simulink model "iros2018_AoA"  (R2017b)
settings: Solver=FixedStepAuto  StartTime=0.0  StopTime=sim_time  FixedStep=1e-5  MaxStep=1e-3  MinStep=1e-19
values from neighbouring files (symbols this model uses):
  g = 9.8    [parameters.m]    (also in parameters.mat)
  I_B = [I_B_x 0 0; 0 I_B_y 0; 0 0 I_B_z]    [parameters.m]    (also in parameters.mat = [5e-10  0  0; 0  5e-10  0; 0  0  1e-09])
  m = 60e-6    (= 6e-05)    [parameters.m]    (also in parameters.mat)
  M2 = [0                  sin(angle)      0               -sin(angle) ... (first row only)    [parameters.m]    (also in parameters.mat = [0 0 1 0 -0.01 0.01 0 0 1 0 -0.01 -0.01 ... (24 elements, 6x)
  M_pitch = -1*[1,1,-1,-1]'    [parameters.m]    (also in parameters.mat = [-1 -1 1 1])
  M_roll = [1,-1,-1,1]'    [parameters.m]    (also in parameters.mat = [1 -1 -1 1])
  M_z = [1,1,1,1]'    [parameters.m]    (also in parameters.mat = [1 1 1 1])
  quad = struct('g',g,'M',m)    [LinearDroneAndPolePlaceControl_ME231b.m]    (also in PolePlacement_DesiredState.m)
  state_des = [0; 0; -.1 ; 0; .00; .00; 0; 0; 0; 0; 0; 0]    [LinearDroneAndPolePlaceControl_ME231b.m]    (also in PolePlacement_DesiredState.m = [0; 0; .015; 0; .00; .00; 0; 0; 0; 0; 0; 0])
  XYZ_initial_condition = [0.0; 0.0; 0.0]    [LinearDroneAndPolePlaceControl_ME231b.m]    (also in PolePlacement_DesiredState.m)
libraries: simulink x15, aerolibutil x2
settings Model: Creator=cbschindler  LastModifiedBy=nato
settings SolverCC: MaxConsecutiveMinStep=15  SolverResetMethod=Robust
settings DataIOCC: LimitDataPoints=on  SaveFormat=Array
settings OptimizationCC: LifeSpan=inf
settings DebuggingCC: ModelReferenceExtraNoncontSigs=none  SFUnexpectedBacktrackingDiag=warning  SFNoUnconditionalDefaultTransitionDiag=warning  SFExecutionAtInitializationDiag=none
settings HardwareCC: ProdBitPerPointer=32  ProdBitPerSizeT=32  ProdBitPerPtrDiffT=32  ProdLargestAtomicFloat=None  ProdIntDivRoundTo=Undefined  ProdEndianess=Unspecified  ProdWordSize=32  ProdHWDeviceType=32-bit Generic
settings ModelReferenceCC: PropagateSignalLabelsOutOfModel=off
settings CodeAppCC: StateflowObjectComments=on
settings GRTTargetCC: TargetLangStandard=C89/C90 (ANSI)  GeneratePreprocessorConditionals=Disable all
settings ConfigComp: CovMetricSettings=dw  CovHtmlReporting=on  CovSaveCumulativeToWorkspaceVar=on  CovSaveSingleToWorkspaceVar=on  CovExternalEMLEnable=off

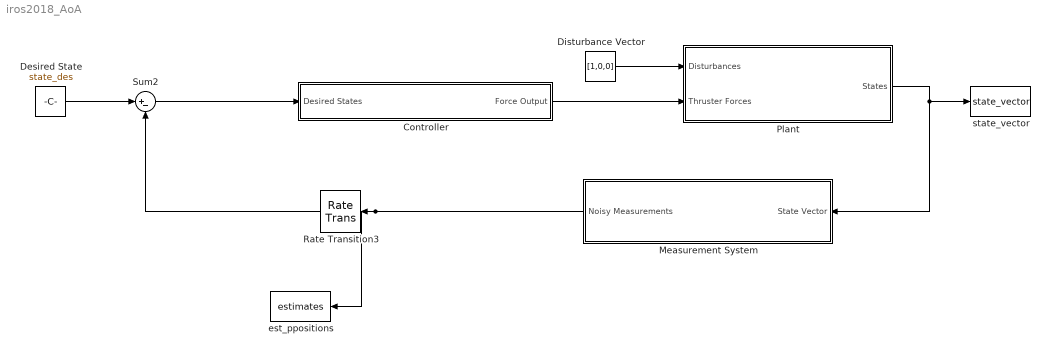
== system iros2018_AoA ==
  Controller : Subsystem
  Desired State : Constant  Value=state_des
  Disturbance Vector : Constant  Value=[1,0,0]
  Measurement System : Subsystem
  Plant : Subsystem
  Rate Transition3 : RateTransition  OutPortSampleTime=0.005
  Sum2 : Sum  Inputs=|+-
  est_ppositions : ToWorkspace  VariableName=estimates  SaveFormat=Timeseries  SampleTime=-1
  state_vector : ToWorkspace  VariableName=state_vector  SaveFormat=Timeseries  SampleTime=-1
  wires:
  Desired State/1 -> Sum2/1
  Rate Transition3/1 -> Sum2/2
  Measurement System/1(Noisy Measurements) -> est_ppositions/1, Rate Transition3/1
  Sum2/1 -> Controller/1(Desired States)
  Plant/1("States ") -> state_vector/1, Measurement System/1("State Vector ")
  Controller/1(Force Output) -> Plant/2(Thruster Forces)
  Disturbance Vector/1 -> Plant/1(Disturbances)

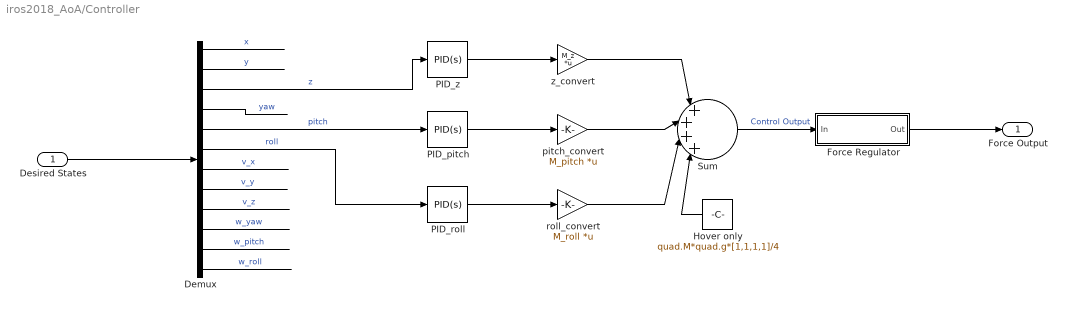
== system iros2018_AoA/Controller ==
  Desired States : Inport
  Demux : Demux  Outputs=12
  Force Regulator : Subsystem
  Hover only : Constant  Value=quad.M*quad.g*[1,1,1,1]/4
  PID_pitch : simulink/Continuous/PID Controller  Controller=PID  TimeDomain=Continuous-time  SampleTime=-1  IntegratorMethod=Forward Euler  FilterMethod=Forward Euler  Form=Parallel  UseFilter=on  ControllerParametersSource=internal  P=0.00000843627433781939  I=.00000750505503699886  D=9.57966094473437e-07  N=33.5514195440974  InitialConditionSource=internal  InitialConditionForIntegrator=0  InitialConditionForFilter=0  ExternalReset=none  LimitOutput=off  UpperSaturationLimit=inf  LowerSaturationLimit=-inf  LinearizeAsGain=on  AntiWindupMode=none  Kb=1  TrackingMode=off  Kt=1  PParamMin=[]  PParamMax=[]  IParamMin=[]  IParamMax=[]  DParamMin=[]  DParamMax=[]  NParamMin=[]  NParamMax=[]  KbParamMin=[]  KbParamMax=[]  KtParamMin=[]  KtParamMax=[]  POutMin=[]  POutMax=[]  IOutMin=[]  IOutMax=[]  DOutMin=[]  DOutMax=[]  NOutMin=[]  NOutMax=[]  KbOutMin=[]  KbOutMax=[]  KtOutMin=[]  KtOutMax=[]  IntegratorOutMin=[]  IntegratorOutMax=[]  FilterOutMin=[]  FilterOutMax=[]  SumOutMin=[]  SumOutMax=[]  SumI1OutMin=[]  SumI1OutMax=[]  SumI2OutMin=[]  SumI2OutMax=[]  SumI3OutMin=[]  SumI3OutMax=[]  SumDOutMin=[]  SumDOutMax=[]  SaturationOutMin=[]  SaturationOutMax=[]  IntegratorContinuousStateAttributes=''  IntegratorStateMustResolveToSignalObject=off  IntegratorRTWStateStorageClass=Auto  FilterContinuousStateAttributes=''  FilterStateMustResolveToSignalObject=off  FilterRTWStateStorageClass=Auto  DifferentiatorICPrevScaledInput=0  DifferentiatorOutMin=[]  DifferentiatorOutMax=[]  InitialConditionSetting=State (most efficient)  FilterDiffOutCoefMin=[]  FilterDiffOutCoefMax=[]  SumDenOutMin=[]  SumDenOutMax=[]  SumNumOutMin=[]  SumNumOutMax=[]  ReciprocalOutMin=[]  ReciprocalOutMax=[]  DivideOutMin=[]  DivideOutMax=[]  TunerSelectOption=Transfer Function Based (PID Tuner App)
  PID_roll : simulink/Continuous/PID Controller  Controller=PID  TimeDomain=Continuous-time  SampleTime=-1  IntegratorMethod=Forward Euler  FilterMethod=Forward Euler  Form=Parallel  UseFilter=on  ControllerParametersSource=internal  P=0.00000843627433781939  I=.00000750505503699886  D=9.57966094473437e-07  N=33.5514195440974  InitialConditionSource=internal  InitialConditionForIntegrator=0  InitialConditionForFilter=0  ExternalReset=none  LimitOutput=off  UpperSaturationLimit=inf  LowerSaturationLimit=-inf  LinearizeAsGain=on  AntiWindupMode=none  Kb=1  TrackingMode=off  Kt=1  PParamMin=[]  PParamMax=[]  IParamMin=[]  IParamMax=[]  DParamMin=[]  DParamMax=[]  NParamMin=[]  NParamMax=[]  KbParamMin=[]  KbParamMax=[]  KtParamMin=[]  KtParamMax=[]  POutMin=[]  POutMax=[]  IOutMin=[]  IOutMax=[]  DOutMin=[]  DOutMax=[]  NOutMin=[]  NOutMax=[]  KbOutMin=[]  KbOutMax=[]  KtOutMin=[]  KtOutMax=[]  IntegratorOutMin=[]  IntegratorOutMax=[]  FilterOutMin=[]  FilterOutMax=[]  SumOutMin=[]  SumOutMax=[]  SumI1OutMin=[]  SumI1OutMax=[]  SumI2OutMin=[]  SumI2OutMax=[]  SumI3OutMin=[]  SumI3OutMax=[]  SumDOutMin=[]  SumDOutMax=[]  SaturationOutMin=[]  SaturationOutMax=[]  IntegratorContinuousStateAttributes=''  IntegratorStateMustResolveToSignalObject=off  IntegratorRTWStateStorageClass=Auto  FilterContinuousStateAttributes=''  FilterStateMustResolveToSignalObject=off  FilterRTWStateStorageClass=Auto  DifferentiatorICPrevScaledInput=0  DifferentiatorOutMin=[]  DifferentiatorOutMax=[]  InitialConditionSetting=State (most efficient)  FilterDiffOutCoefMin=[]  FilterDiffOutCoefMax=[]  SumDenOutMin=[]  SumDenOutMax=[]  SumNumOutMin=[]  SumNumOutMax=[]  ReciprocalOutMin=[]  ReciprocalOutMax=[]  DivideOutMin=[]  DivideOutMax=[]  TunerSelectOption=Transfer Function Based (PID Tuner App)
  PID_z : simulink/Continuous/PID Controller  Controller=PID  TimeDomain=Continuous-time  SampleTime=-1  IntegratorMethod=Forward Euler  FilterMethod=Forward Euler  Form=Parallel  UseFilter=on  ControllerParametersSource=internal  P=0.00000843627433781939  I=0.00000750505503699886  D=9.57966094473437e-07  N=.335514195440974  InitialConditionSource=internal  InitialConditionForIntegrator=0  InitialConditionForFilter=0  ExternalReset=none  LimitOutput=off  UpperSaturationLimit=inf  LowerSaturationLimit=-inf  LinearizeAsGain=on  AntiWindupMode=none  Kb=1  TrackingMode=off  Kt=1  PParamMin=[]  PParamMax=[]  IParamMin=[]  IParamMax=[]  DParamMin=[]  DParamMax=[]  NParamMin=[]  NParamMax=[]  KbParamMin=[]  KbParamMax=[]  KtParamMin=[]  KtParamMax=[]  POutMin=[]  POutMax=[]  IOutMin=[]  IOutMax=[]  DOutMin=[]  DOutMax=[]  NOutMin=[]  NOutMax=[]  KbOutMin=[]  KbOutMax=[]  KtOutMin=[]  KtOutMax=[]  IntegratorOutMin=[]  IntegratorOutMax=[]  FilterOutMin=[]  FilterOutMax=[]  SumOutMin=[]  SumOutMax=[]  SumI1OutMin=[]  SumI1OutMax=[]  SumI2OutMin=[]  SumI2OutMax=[]  SumI3OutMin=[]  SumI3OutMax=[]  SumDOutMin=[]  SumDOutMax=[]  SaturationOutMin=[]  SaturationOutMax=[]  IntegratorContinuousStateAttributes=''  IntegratorStateMustResolveToSignalObject=off  IntegratorRTWStateStorageClass=Auto  FilterContinuousStateAttributes=''  FilterStateMustResolveToSignalObject=off  FilterRTWStateStorageClass=Auto  DifferentiatorICPrevScaledInput=0  DifferentiatorOutMin=[]  DifferentiatorOutMax=[]  InitialConditionSetting=State (most efficient)  FilterDiffOutCoefMin=[]  FilterDiffOutCoefMax=[]  SumDenOutMin=[]  SumDenOutMax=[]  SumNumOutMin=[]  SumNumOutMax=[]  ReciprocalOutMin=[]  ReciprocalOutMax=[]  DivideOutMin=[]  DivideOutMax=[]  TunerSelectOption=Transfer Function Based (PID Tuner App)
  Sum : Sum  Inputs=|++++|
  pitch_convert : Gain  Gain=M_pitch  Multiplication=Matrix(K*u)
  roll_convert : Gain  Gain=M_roll  Multiplication=Matrix(K*u)
  z_convert : Gain  Gain=M_z  Multiplication=Matrix(K*u)
  Force Output : Outport
  wires:
  Desired States/1 -> Demux/1
  Force Regulator/1(Out) -> Force Output/1
  Demux/1 -> ?  "x"
  Demux/2 -> ?  "y"
  Demux/3 -> PID_z/1  "z"
  Demux/4 -> ?  "yaw"
  PID_z/1 -> z_convert/1
  Demux/5 -> PID_pitch/1  "pitch"
  Demux/6 -> PID_roll/1  "roll"
  Demux/7 -> ?  "v_x"
  Demux/8 -> ?  "v_y"
  Demux/9 -> ?  "v_z"
  Demux/10 -> ?  "w_yaw"
  Demux/11 -> ?  "w_pitch"
  Demux/12 -> ?  "w_roll"
  z_convert/1 -> Sum/1
  PID_pitch/1 -> pitch_convert/1
  pitch_convert/1 -> Sum/2
  roll_convert/1 -> Sum/3
  Sum/1 -> Force Regulator/1(In)  "Control Output"
  PID_roll/1 -> roll_convert/1
  Hover only/1 -> Sum/4

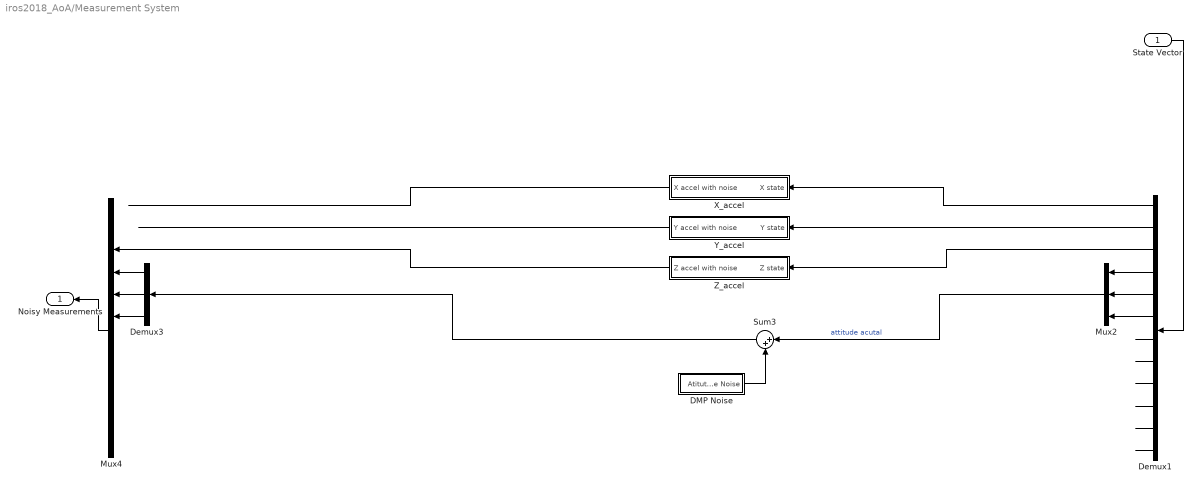
== system iros2018_AoA/Measurement System ==
  "State Vector " : Inport
  DMP Noise : Subsystem
  Demux1 : Demux  Outputs=12
  Demux3 : Demux  Outputs=3
  Mux2 : Mux  Inputs=3
  Mux4 : Mux  Inputs=12
  Sum3 : Sum  Inputs=|++
  X_accel : Subsystem
  Y_accel : Subsystem
  Z_accel : Subsystem
  Noisy Measurements : Outport
  wires:
  Demux1/4 -> Mux2/1
  Demux1/5 -> Mux2/2
  Demux1/6 -> Mux2/3
  Sum3/1 -> Demux3/1
  Demux3/1 -> Mux4/4
  Demux3/2 -> Mux4/5
  Demux3/3 -> Mux4/6
  Mux4/1 -> Noisy Measurements/1
  Demux1/1 -> X_accel/1(X state)
  Demux1/2 -> Y_accel/1(Y state)
  X_accel/1(X accel with noise) -> ?
  "State Vector "/1 -> Demux1/1
  ? -> Mux4/12
  Demux1/7 -> ?
  ? -> Mux4/9
  Demux1/10 -> ?
  Demux1/11 -> ?
  Y_accel/1(Y accel with noise) -> ?
  Demux1/9 -> ?
  ? -> Mux4/10
  Demux1/12 -> ?
  Demux1/8 -> ?
  ? -> Mux4/7
  ? -> Mux4/8
  ? -> Mux4/11
  Mux2/1 -> Sum3/1  "attitude acutal"
  DMP Noise/1(Atitutude Noise) -> Sum3/2
  Demux1/3 -> Z_accel/1(Z state)
  Z_accel/1(Z accel with noise) -> Mux4/3

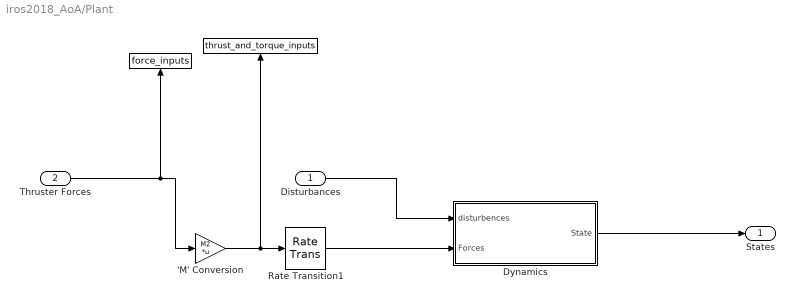
== system iros2018_AoA/Plant ==
  Disturbances : Inport
  Thruster Forces : Inport  Port=2
  " " : ToWorkspace  VariableName=force_inputs  SaveFormat=Timeseries  SampleTime=-1
  "  " : ToWorkspace  VariableName=thrust_and_torque_inputs  SaveFormat=Timeseries  SampleTime=-1
  'M' Conversion : Gain  Gain=M2  Multiplication=Matrix(K*u)
  Dynamics : Subsystem
  Rate Transition1 : RateTransition  OutPortSampleTime=1e-5
  "States " : Outport
  wires:
  'M' Conversion/1 -> Rate Transition1/1, "  "/1
  Dynamics/1(State) -> "States "/1
  Rate Transition1/1 -> Dynamics/2(Forces)
  Thruster Forces/1 -> " "/1, 'M' Conversion/1
  Disturbances/1 -> Dynamics/1(disturbences)

== system iros2018_AoA/Controller/Force Regulator ==
  In : Inport
  Force Correction : Subsystem
  Max Iono Force (N) : Constant  Value=3e-4
  Out : Outport
  wires:
  Max Iono Force (N)/1 -> Force Correction/2(Max Force)
  In/1 -> Force Correction/1(Input)
  Force Correction/1(Output) -> Out/1  "Adjusted Thruster Fors"

== system iros2018_AoA/Measurement System/DMP Noise ==
  Mux : Mux  Inputs=3
  Scope : Scope
  pitch_noise : simulink/Sources/Band-Limited White Noise  Cov=2.5e-8  Ts=1e-5  seed=[7686]  VectorParams1D=off
  roll_noise : simulink/Sources/Band-Limited White Noise  Cov=2.5e-8  Ts=1e-5  seed=[1231]  VectorParams1D=off
  yaw_noise : simulink/Sources/Band-Limited White Noise  Cov=1e-7  Ts=1e-5  seed=[45645]  VectorParams1D=off
  Atitutude Noise : Outport
  wires:
  pitch_noise/1 -> Mux/2
  Mux/1 -> Scope/1, Atitutude Noise/1
  yaw_noise/1 -> Mux/1
  roll_noise/1 -> Mux/3

== system iros2018_AoA/Measurement System/X_accel ==
  X state : Inport
  Discrete Derivative : simulink/Discrete/Discrete Derivative  gainval=1.0  ICPrevScaledInput=0.0  OutMin=[]  OutMax=[]  OutDataType=fixdt(1, 16)  OutScaling=2^-10  DoSatur=off
  Discrete Derivative1 : simulink/Discrete/Discrete Derivative  gainval=1.0  ICPrevScaledInput=0.0  OutMin=[]  OutMax=[]  OutDataType=fixdt(1, 16)  OutScaling=2^-10  DoSatur=off
  Sum4 : Sum  Inputs=++|
  accel : ToWorkspace  VariableName=accel_x  SaveFormat=Timeseries  SampleTime=-1
  acceleromter noise : Subsystem
  X accel with noise : Outport
  wires:
  X state/1 -> Discrete Derivative/1
  acceleromter noise/1(noise) -> Sum4/1
  Sum4/1 -> X accel with noise/1
  Discrete Derivative/1 -> Discrete Derivative1/1
  Discrete Derivative1/1 -> Sum4/2, accel/1

== system iros2018_AoA/Measurement System/Y_accel ==
  Y state : Inport
  Discrete Derivative : simulink/Discrete/Discrete Derivative  gainval=1.0  ICPrevScaledInput=0.0  OutMin=[]  OutMax=[]  OutDataType=fixdt(1, 16)  OutScaling=2^-10  DoSatur=off
  Discrete Derivative1 : simulink/Discrete/Discrete Derivative  gainval=1.0  ICPrevScaledInput=0.0  OutMin=[]  OutMax=[]  OutDataType=fixdt(1, 16)  OutScaling=2^-10  DoSatur=off
  Sum4 : Sum  Inputs=++|
  accel : ToWorkspace  VariableName=accel_y  SaveFormat=Timeseries  SampleTime=-1
  acceleromter noise : Subsystem
  Y accel with noise : Outport
  wires:
  Y state/1 -> Discrete Derivative/1
  acceleromter noise/1(noise) -> Sum4/1
  Sum4/1 -> Y accel with noise/1
  Discrete Derivative/1 -> Discrete Derivative1/1
  Discrete Derivative1/1 -> Sum4/2, accel/1

== system iros2018_AoA/Measurement System/Z_accel ==
  Z state : Inport
  Discrete Derivative : simulink/Discrete/Discrete Derivative  gainval=1.0  ICPrevScaledInput=0.0  OutMin=[]  OutMax=[]  OutDataType=fixdt(1, 16)  OutScaling=2^-10  DoSatur=off
  Discrete Derivative1 : simulink/Discrete/Discrete Derivative  gainval=1.0  ICPrevScaledInput=0.0  OutMin=[]  OutMax=[]  OutDataType=fixdt(1, 16)  OutScaling=2^-10  DoSatur=off
  Sum4 : Sum  Inputs=++|
  accel : ToWorkspace  VariableName=accel_z  SaveFormat=Timeseries  SampleTime=-1
  acceleromter noise : Subsystem
  Z accel with noise : Outport
  wires:
  Z state/1 -> Discrete Derivative/1
  acceleromter noise/1(noise) -> Sum4/1
  Sum4/1 -> Z accel with noise/1
  Discrete Derivative/1 -> Discrete Derivative1/1
  Discrete Derivative1/1 -> Sum4/2, accel/1

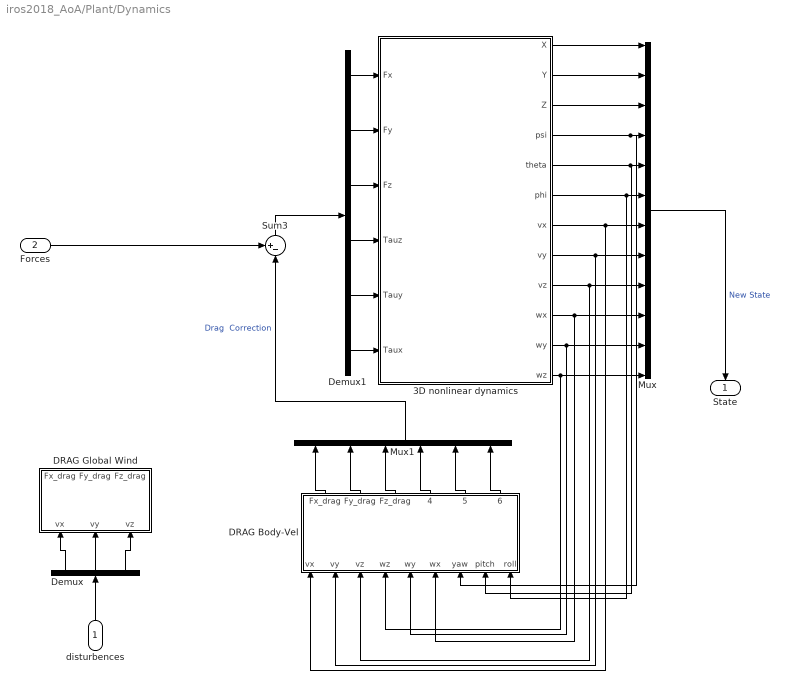
== system iros2018_AoA/Plant/Dynamics ==
  disturbences : Inport
  Forces : Inport  Port=2
  3D nonlinear dynamics : Subsystem
  DRAG Body-Vel : Subsystem
  DRAG Global Wind : Subsystem
  Demux : Demux  Outputs=3
  Demux1 : Demux  Outputs=6
  Mux : Mux  Inputs=12
  Mux1 : Mux  Inputs=6
  Sum3 : Sum  Inputs=+-|
  State : Outport
  wires:
  DRAG Body-Vel/1(Fx_drag) -> Mux1/1
  Sum3/1 -> Demux1/1
  Mux1/1 -> Sum3/2  "Drag  Correction"
  Mux/1 -> State/1  "New State"
  3D nonlinear dynamics/7(vx) -> Mux/7, DRAG Body-Vel/1(vx)
  Demux1/6 -> 3D nonlinear dynamics/6(Taux)
  3D nonlinear dynamics/8(vy) -> Mux/8, DRAG Body-Vel/2(vy)
  Demux1/2 -> 3D nonlinear dynamics/2(Fy)
  Demux1/1 -> 3D nonlinear dynamics/1(Fx)
  Demux1/4 -> 3D nonlinear dynamics/4(Tauz)
  Demux1/5 -> 3D nonlinear dynamics/5(Tauy)
  3D nonlinear dynamics/9(vz) -> Mux/9, DRAG Body-Vel/3(vz)
  3D nonlinear dynamics/10(wx) -> Mux/10, DRAG Body-Vel/6(wx)
  Demux1/3 -> 3D nonlinear dynamics/3(Fz)
  3D nonlinear dynamics/11(wy) -> Mux/11, DRAG Body-Vel/5(wy)
  3D nonlinear dynamics/12(wz) -> Mux/12, DRAG Body-Vel/4(wz)
  3D nonlinear dynamics/1(X) -> Mux/1
  3D nonlinear dynamics/2(Y) -> Mux/2
  3D nonlinear dynamics/3(Z) -> Mux/3
  3D nonlinear dynamics/4(psi) -> Mux/4, DRAG Body-Vel/7(yaw)
  3D nonlinear dynamics/5(theta) -> DRAG Body-Vel/8(pitch), Mux/5
  3D nonlinear dynamics/6(phi) -> Mux/6, DRAG Body-Vel/9("roll ")
  DRAG Body-Vel/3(Fz_drag) -> Mux1/3
  DRAG Body-Vel/5(Tauy_drag) -> Mux1/5
  DRAG Body-Vel/6(Taux_drag) -> Mux1/6
  DRAG Body-Vel/4(Tauz_drag) -> Mux1/4
  DRAG Body-Vel/2(Fy_drag) -> Mux1/2
  disturbences/1 -> Demux/1
  Forces/1 -> Sum3/1
  Demux/1 -> DRAG Global Wind/1(vx)
  Demux/2 -> DRAG Global Wind/2(vy)
  Demux/3 -> DRAG Global Wind/3(vz)

== system iros2018_AoA/Controller/Force Regulator/Force Correction ==
  Input : Inport
  Max Force : Inport  Port=2
  Clock : Clock
  MATLAB Function : MATLAB Function  TreatAsAtomicUnit=on
  Output : Outport
  wires:
  Input/1 -> MATLAB Function/1(u)
  MATLAB Function/1(y) -> Output/1
  Max Force/1 -> MATLAB Function/2(maxF)
  Clock/1 -> MATLAB Function/3(t)

== system iros2018_AoA/Measurement System/X_accel/acceleromter noise ==
  z_noise : simulink/Sources/Band-Limited White Noise  Cov=300*9.8e-6  Ts=1e-5  seed=[23341]  VectorParams1D=off
  noise : Outport
  wires:
  z_noise/1 -> noise/1

== system iros2018_AoA/Measurement System/Y_accel/acceleromter noise ==
  z_noise : simulink/Sources/Band-Limited White Noise  Cov=300*9.8e-6  Ts=1e-5  seed=[23341]  VectorParams1D=off
  noise : Outport
  wires:
  z_noise/1 -> noise/1

== system iros2018_AoA/Measurement System/Z_accel/acceleromter noise ==
  z_noise : simulink/Sources/Band-Limited White Noise  Cov=300*9.8e-6  Ts=1e-5  seed=[23341]  VectorParams1D=off
  noise : Outport
  wires:
  z_noise/1 -> noise/1

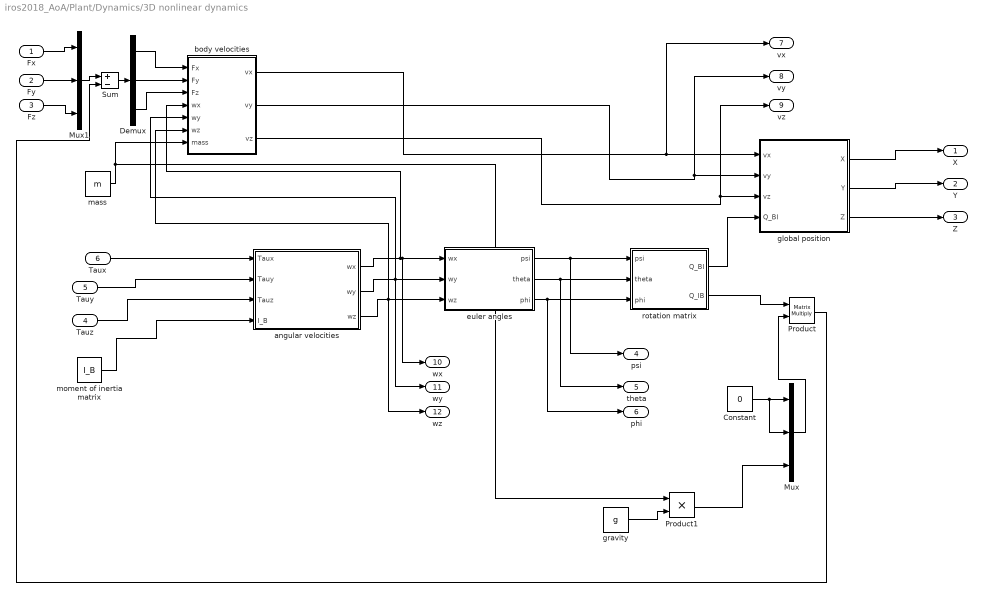
== system iros2018_AoA/Plant/Dynamics/3D nonlinear dynamics ==
  Fx : Inport
  Fy : Inport  Port=2
  Fz : Inport  Port=3
  Tauz : Inport  Port=4
  Tauy : Inport  Port=5
  Taux : Inport  Port=6
  Constant : Constant  Value=0
  Demux : Demux  Outputs=3
  Mux : Mux  Inputs=3
  Mux1 : Mux  Inputs=3
  Product : Product  Multiplication=Matrix(*)
  Product1 : Product
  Sum : Sum  Inputs=+-
  angular velocities : Subsystem
  body velocities : Subsystem
  euler angles : Subsystem
  global position : Subsystem
  gravity : Constant  Value=g
  mass : Constant  Value=m
  moment of inertia matrix : Constant  Value=I_B
  rotation matrix : Subsystem
  X : Outport
  Y : Outport  Port=2
  Z : Outport  Port=3
  psi : Outport  Port=4
  theta : Outport  Port=5
  phi : Outport  Port=6
  vx : Outport  Port=7
  vy : Outport  Port=8
  vz : Outport  Port=9
  wx : Outport  Port=10
  wy : Outport  Port=11
  wz : Outport  Port=12
  wires:
  angular velocities/3(wz) -> euler angles/3(wz), body velocities/6(wz), wz/1
  Demux/3 -> body velocities/3(Fz)
  global position/3(Z) -> Z/1
  Fy/1 -> Mux1/2
  Fz/1 -> Mux1/3
  body velocities/2(vy) -> global position/2(vy), vy/1
  euler angles/1(psi) -> rotation matrix/1(psi), psi/1
  Demux/2 -> body velocities/2(Fy)
  Mux/1 -> Product/2
  mass/1 -> body velocities/7(mass), Product1/1
  Constant/1 -> Mux/1, Mux/2
  euler angles/3(phi) -> rotation matrix/3(phi), phi/1
  Mux1/1 -> Sum/1
  Product/1 -> Sum/2
  body velocities/3(vz) -> global position/3(vz), vz/1
  moment of inertia matrix/1 -> angular velocities/4(I_B)
  angular velocities/2(wy) -> euler angles/2(wy), body velocities/5(wy), wy/1
  Sum/1 -> Demux/1
  Product1/1 -> Mux/3
  Tauy/1 -> angular velocities/2(Tauy)
  global position/2(Y) -> Y/1
  Demux/1 -> body velocities/1(Fx)
  rotation matrix/2(Q_IB) -> Product/1
  rotation matrix/1(Q_BI) -> global position/4(Q_BI)
  body velocities/1(vx) -> global position/1(vx), vx/1
  gravity/1 -> Product1/2
  Fx/1 -> Mux1/1
  global position/1(X) -> X/1
  euler angles/2(theta) -> rotation matrix/2(theta), theta/1
  angular velocities/1(wx) -> body velocities/4(wx), euler angles/1(wx), wx/1
  Tauz/1 -> angular velocities/3(Tauz)
  Taux/1 -> angular velocities/1(Taux)

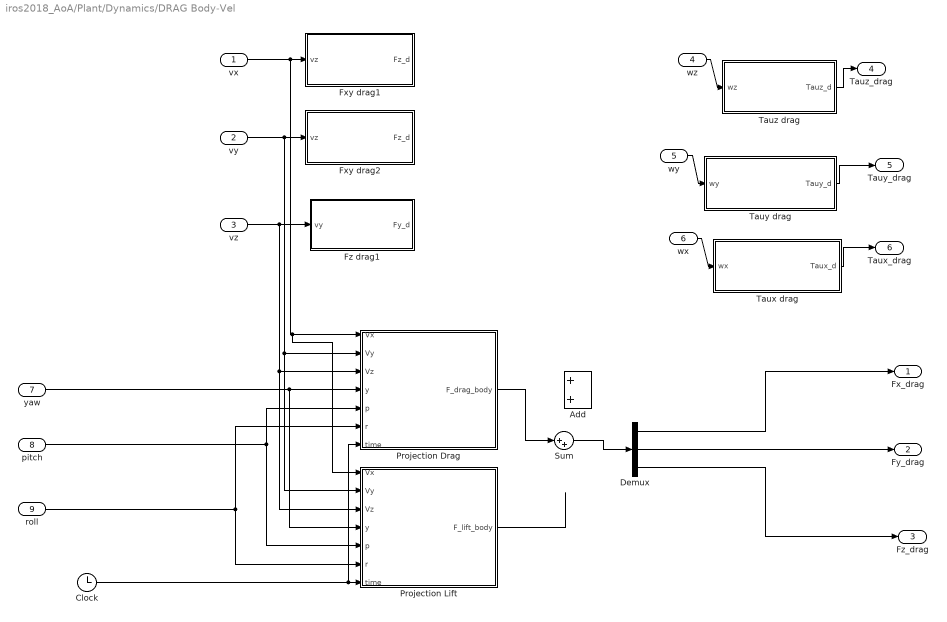
== system iros2018_AoA/Plant/Dynamics/DRAG Body-Vel ==
  vx : Inport
  vy : Inport  Port=2
  vz : Inport  Port=3
  wz : Inport  Port=4
  wy : Inport  Port=5
  wx : Inport  Port=6
  yaw : Inport  Port=7
  pitch : Inport  Port=8
  "roll " : Inport  Port=9
  Add : Sum
  Clock : Clock
  Demux : Demux  Outputs=3
  Fxy drag1 : MATLAB Function  TreatAsAtomicUnit=on
  Fxy drag2 : MATLAB Function  TreatAsAtomicUnit=on
  Fz drag1 : MATLAB Function  TreatAsAtomicUnit=on
  Projection Drag : MATLAB Function  TreatAsAtomicUnit=on
  Projection Lift : MATLAB Function  TreatAsAtomicUnit=on
  Sum : Sum  Inputs=|++
  Taux drag : MATLAB Function  TreatAsAtomicUnit=on
  Tauy drag : MATLAB Function  TreatAsAtomicUnit=on
  Tauz drag : MATLAB Function  TreatAsAtomicUnit=on
  Fx_drag : Outport
  Fy_drag : Outport  Port=2
  Fz_drag : Outport  Port=3
  Tauz_drag : Outport  Port=4
  Tauy_drag : Outport  Port=5
  Taux_drag : Outport  Port=6
  wires:
  vx/1 -> Projection Lift/1(Vx), Projection Drag/1(Vx), Fxy drag1/1(vz)
  vy/1 -> Projection Lift/2(Vy), Projection Drag/2(Vy), Fxy drag2/1(vz)
  vz/1 -> Projection Lift/3(Vz), Projection Drag/3(Vz), Fz drag1/1(vy)
  Tauz drag/1(Tauz_d) -> Tauz_drag/1
  wz/1 -> Tauz drag/1(wz)
  Tauy drag/1(Tauy_d) -> Tauy_drag/1
  wy/1 -> Tauy drag/1(wy)
  Taux drag/1(Taux_d) -> Taux_drag/1
  wx/1 -> Taux drag/1(wx)
  Projection Drag/1(F_drag_body) -> Sum/1
  yaw/1 -> Projection Lift/4(y), Projection Drag/4(y)
  pitch/1 -> Projection Drag/5(p), Projection Lift/5(p)
  "roll "/1 -> Projection Drag/6(r), Projection Lift/6(r)
  Demux/1 -> Fx_drag/1
  Demux/2 -> Fy_drag/1
  Demux/3 -> Fz_drag/1
  Clock/1 -> Projection Drag/7(time), Projection Lift/7(time)
  Projection Lift/1(F_lift_body) -> ?
  Sum/1 -> Demux/1

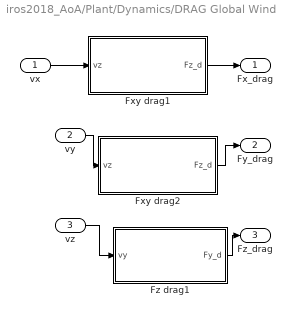
== system iros2018_AoA/Plant/Dynamics/DRAG Global Wind ==
  vx : Inport
  vy : Inport  Port=2
  vz : Inport  Port=3
  Fxy drag1 : MATLAB Function  TreatAsAtomicUnit=on
  Fxy drag2 : MATLAB Function  TreatAsAtomicUnit=on
  Fz drag1 : MATLAB Function  TreatAsAtomicUnit=on
  Fx_drag : Outport
  Fy_drag : Outport  Port=2
  Fz_drag : Outport  Port=3
  wires:
  Fxy drag1/1(Fz_d) -> Fx_drag/1
  vx/1 -> Fxy drag1/1(vz)
  Fxy drag2/1(Fz_d) -> Fy_drag/1
  vy/1 -> Fxy drag2/1(vz)
  Fz drag1/1(Fy_d) -> Fz_drag/1
  vz/1 -> Fz drag1/1(vy)

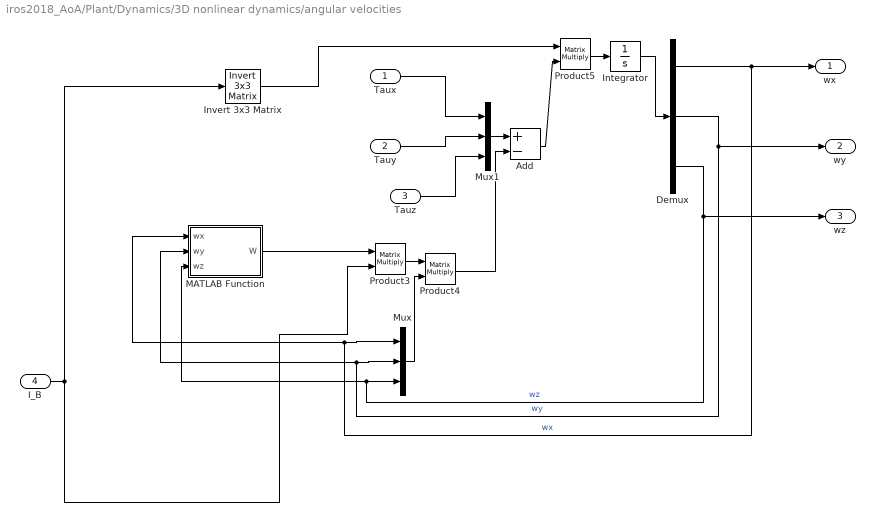
== system iros2018_AoA/Plant/Dynamics/3D nonlinear dynamics/angular velocities ==
  Taux : Inport
  Tauy : Inport  Port=2
  Tauz : Inport  Port=3
  I_B : Inport  Port=4
  Add : Sum  Inputs=+-
  Demux : Demux  Outputs=3
  Integrator : Integrator
  Invert 3x3 Matrix : aerolibutil/Invert  3x3 Matrix
  MATLAB Function : MATLAB Function  TreatAsAtomicUnit=on
  Mux : Mux  Inputs=3
  Mux1 : Mux  Inputs=3
  Product3 : Product  Multiplication=Matrix(*)
  Product4 : Product  Multiplication=Matrix(*)
  Product5 : Product  Multiplication=Matrix(*)
  wx : Outport
  wy : Outport  Port=2
  wz : Outport  Port=3
  wires:
  Product4/1 -> Add/2
  Integrator/1 -> Demux/1
  Invert 3x3 Matrix/1 -> Product5/1
  Product5/1 -> Integrator/1
  Demux/2 -> wy/1, Mux/2, MATLAB Function/2(wy)  "wy"
  I_B/1 -> Invert 3x3 Matrix/1, Product3/2
  Taux/1 -> Mux1/1
  Demux/1 -> wx/1, Mux/1, MATLAB Function/1(wx)  "wx"
  MATLAB Function/1(W) -> Product3/1
  Tauz/1 -> Mux1/3
  Product3/1 -> Product4/1
  Tauy/1 -> Mux1/2
  Mux1/1 -> Add/1
  Mux/1 -> Product4/2
  Add/1 -> Product5/2
  Demux/3 -> wz/1, Mux/3, MATLAB Function/3(wz)  "wz"

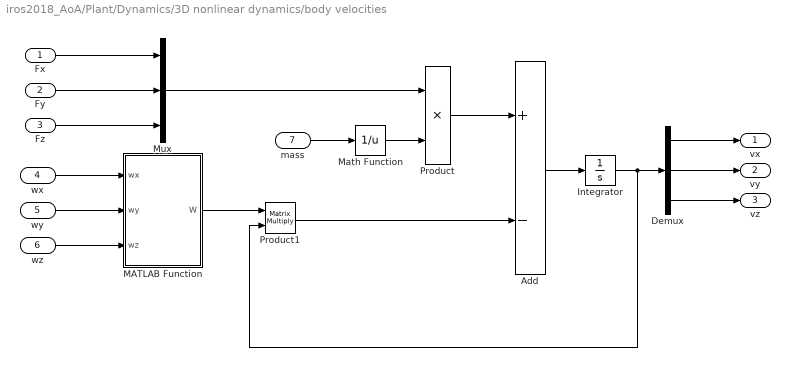
== system iros2018_AoA/Plant/Dynamics/3D nonlinear dynamics/body velocities ==
  Fx : Inport
  Fy : Inport  Port=2
  Fz : Inport  Port=3
  wx : Inport  Port=4
  wy : Inport  Port=5
  wz : Inport  Port=6
  mass : Inport  Port=7
  Add : Sum  Inputs=+-
  Demux : Demux  Outputs=3
  Integrator : Integrator
  MATLAB Function : MATLAB Function  TreatAsAtomicUnit=on
  Math Function : Math  Operator=reciprocal  SaturateOnIntegerOverflow=on
  Mux : Mux  Inputs=3
  Product : Product
  Product1 : Product  Multiplication=Matrix(*)
  vx : Outport
  vy : Outport  Port=2
  vz : Outport  Port=3
  wires:
  Fx/1 -> Mux/1
  Fy/1 -> Mux/2
  Fz/1 -> Mux/3
  Mux/1 -> Product/1
  Math Function/1 -> Product/2
  Product/1 -> Add/1
  Product1/1 -> Add/2
  Add/1 -> Integrator/1
  Integrator/1 -> Demux/1, Product1/2
  Demux/1 -> vx/1
  Demux/2 -> vy/1
  Demux/3 -> vz/1
  mass/1 -> Math Function/1
  wx/1 -> MATLAB Function/1(wx)
  wy/1 -> MATLAB Function/2(wy)
  wz/1 -> MATLAB Function/3(wz)
  MATLAB Function/1(W) -> Product1/1

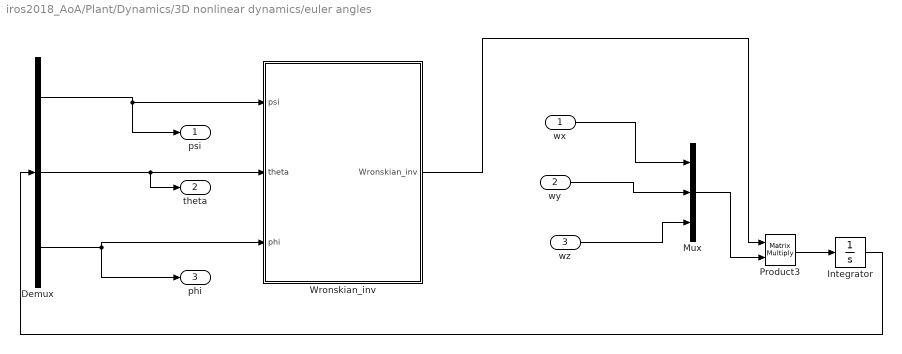
== system iros2018_AoA/Plant/Dynamics/3D nonlinear dynamics/euler angles ==
  wx : Inport
  wy : Inport  Port=2
  wz : Inport  Port=3
  Demux : Demux  Outputs=3
  Integrator : Integrator
  Mux : Mux  Inputs=3
  Product3 : Product  Multiplication=Matrix(*)
  Wronskian_inv : MATLAB Function  TreatAsAtomicUnit=on
  psi : Outport
  theta : Outport  Port=2
  phi : Outport  Port=3
  wires:
  Demux/3 -> phi/1, Wronskian_inv/3(phi)
  Demux/1 -> psi/1, Wronskian_inv/1(psi)
  Demux/2 -> theta/1, Wronskian_inv/2(theta)
  Wronskian_inv/1(Wronskian_inv) -> Product3/1
  wx/1 -> Mux/1
  wy/1 -> Mux/2
  wz/1 -> Mux/3
  Mux/1 -> Product3/2
  Product3/1 -> Integrator/1
  Integrator/1 -> Demux/1

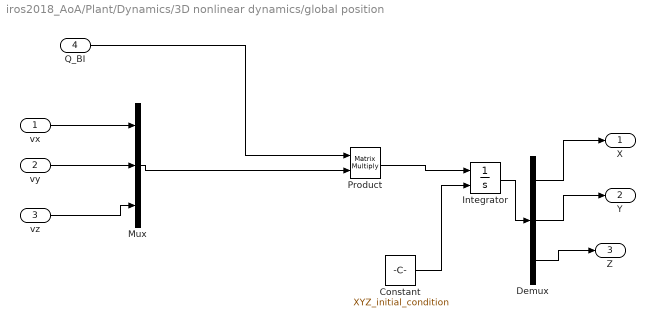
== system iros2018_AoA/Plant/Dynamics/3D nonlinear dynamics/global position ==
  vx : Inport
  vy : Inport  Port=2
  vz : Inport  Port=3
  Q_BI : Inport  Port=4
  Constant : Constant  Value=XYZ_initial_condition
  Demux : Demux  Outputs=3
  Integrator : Integrator  InitialConditionSource=external
  Mux : Mux  Inputs=3
  Product : Product  Multiplication=Matrix(*)
  X : Outport
  Y : Outport  Port=2
  Z : Outport  Port=3
  wires:
  Integrator/1 -> Demux/1
  vz/1 -> Mux/3
  Demux/2 -> Y/1
  Q_BI/1 -> Product/1
  Mux/1 -> Product/2
  Demux/3 -> Z/1
  vy/1 -> Mux/2
  Demux/1 -> X/1
  Product/1 -> Integrator/1
  vx/1 -> Mux/1
  Constant/1 -> Integrator/2

== system iros2018_AoA/Plant/Dynamics/3D nonlinear dynamics/rotation matrix ==
  psi : Inport
  theta : Inport  Port=2
  phi : Inport  Port=3
  MATLAB Function : MATLAB Function  TreatAsAtomicUnit=on
  Q_BI_inv : aerolibutil/Invert  3x3 Matrix
  Q_BI : Outport
  Q_IB : Outport  Port=2
  wires:
  Q_BI_inv/1 -> Q_IB/1
  psi/1 -> MATLAB Function/1(psi)
  phi/1 -> MATLAB Function/3(phi)
  MATLAB Function/1(Q_BI) -> Q_BI/1, Q_BI_inv/1
  theta/1 -> MATLAB Function/2(theta)

== matlab function iros2018_AoA/Plant/Dynamics/3D nonlinear dynamics/angular velocities/MATLAB Function ==
  data: wx input; W output; wy input; wz input
function W = fcn(wx,wy,wz)
%#codegen

W = [0 -wz wy;
     wz 0 -wx;
     -wy wx 0];

== matlab function iros2018_AoA/Plant/Dynamics/3D nonlinear dynamics/body velocities/MATLAB Function ==
  data: wx input; W output; wy input; wz input
function W = fcn(wx,wy,wz)
%#codegen

W = [0 -wz wy;
     wz 0 -wx;
     -wy wx 0];

== matlab function iros2018_AoA/Plant/Dynamics/3D nonlinear dynamics/euler angles/Wronskian_inv ==
  data: psi input; Wronskian_inv output; theta input; phi input
function Wronskian_inv = fcn(psi,theta,phi)
%#codegen

Wronskian_inv = (1/cos(theta)).*[0, sin(phi), cos(phi);
                                 0, cos(phi)*cos(theta), -sin(phi)*cos(theta);
                                 cos(theta), sin(phi)*sin(theta), cos(phi)*sin(theta);];

== matlab function iros2018_AoA/Plant/Dynamics/3D nonlinear dynamics/rotation matrix/MATLAB Function ==
  data: psi input; Q_BI output; theta input; phi input
function Q_BI = fcn(psi, theta, phi)
%#codegen

Q_BI = [cos(theta)*cos(psi), cos(psi)*sin(theta)*sin(phi)-cos(phi)*sin(psi), sin(phi)*sin(psi)+cos(phi)*cos(psi)*sin(theta);
        cos(theta)*sin(psi), cos(phi)*cos(psi)+sin(theta)*sin(phi)*sin(psi), cos(phi)*sin(theta)*sin(psi)-cos(psi)*sin(phi);
        -sin(theta), cos(theta)*sin(phi), cos(theta)*cos(phi)];

== matlab function iros2018_AoA/Plant/Dynamics/DRAG Body-Vel/Projection Drag ==
  data: Vx input; F_drag_body output; Vy input; Vz input; y input; p input; r input; time input
function F_drag_body = fcn(Vx, Vy, Vz, y, p, r, time)
%#codegen
% Takes in body velocity vectors and returns global drag force vector
%       V_body = [vx, vy, vz]
%       Drag_body = f([vx, vy, vz]) 
%       [Fx, Fy, Fz] = f(drag_body, [yaw, pitch, roll])

% Drag is fit to:
%   f(theta,v) = (w1*theta+w2)*v^2+(w3*theta+w4)*v
%   w= [-0.07370093  0.09642926 -0.06727348  0.11939324]

% This approximation is only valid for small angles of attack, so theta is
% in the bounded region of [0,30] ish

% If needed: Fitting body drag vector to global is just the transformation of body to
% global with yaw pitch and roll

%% Grabs values for projections
if time == 0
    F_drag_body = [0,0,0];
else  
    
% Vb
% Vx = Vb(1);
% Vy = Vb(2);
% Vz = Vb(3);

w= [-0.07370093  0.09642926 -0.06727348  0.11939324];

% yaw = attitude(1);
% pitch = attitude(2);
% roll = attitude(3);

% Extracts Angles
theta_yz = atan(Vz/Vy);
theta_xz = atan(Vz/Vx);

% Gets velocity number
v_yz = norm([Vy, Vz]);
v_xz = norm([Vx, Vz]);

% Computes Drag
F_d_yz = (w(1)*(pi/2-theta_yz)+w(2))*v_yz^2 + (w(3)*(pi/2-theta_yz)+w(4))*v_yz^2;
F_d_xz = (w(1)*(pi/2-theta_xz)+w(2))*v_xz^2 + (w(3)*(pi/2-theta_xz)+w(4))*v_xz^2;

% Vectorized drag output

F_d_yz_v = 1e-3.*[0, Vy/(Vy + Vz), .5*Vz/(Vy + Vz)] .* F_d_yz;
F_d_xz_v = 1e-3.*[Vx/(Vx + Vz), 0, .5*Vz/(Vx + Vz)] .* F_d_xz;
%{
%% Defines matrices for getting global forces
Ryaw = [
	[ cos(yaw), -sin(yaw), 0],
	[ sin(yaw),  cos(yaw), 0],
	[        0,         0, 1]
];

Rpitch = [
	[  cos(pitch), 0, sin(pitch)],
	[           0, 1,          0],
	[ -sin(pitch), 0, cos(pitch)]
];

Rroll = [
	[ 1,         0,          0],
	[ 0, cos(roll), -sin(roll)],
	[ 0, sin(roll),  cos(roll)]
];

Body2Global = Ryaw*Rpitch*Rroll;
%}
% F_drag_body = [0, 0, 0];
F_drag_body = [F_d_xz_v(1), F_d_yz_v(2), F_d_xz_v(3)+F_d_yz_v(3)];

end 
% F_drag = Body2Global*F_drag_body;

== matlab function iros2018_AoA/Plant/Dynamics/DRAG Body-Vel/Fxy drag1 ==
  data: vz input; Fz_d output
function Fz_d = fcn(vz)
%#codegen
% v = max( 0.001,min(1,vz));
% i = round(v*1000);
% Fz_d = Fz_drag(i);
% fitFz = 
% 
%      General model:
%      fitFz(x) = a*x^2 + b*x
%      Coefficients (with 95% confidence bounds):
%        a =   4.315e-07  (4.307e-07, 4.324e-07)
%        b =   1.147e-06  (1.143e-06, 1.15e-06)    

if (vz >=0)
    Fz_d = 4.315e-07.*vz.^2+1.147e-06.*vz;%+-1.59e-07;
else
    Fz_d = -(4.315e-07.*vz.^2)+1.147e-06.*vz;%+-1.59e-07;
end

== matlab function iros2018_AoA/Plant/Dynamics/DRAG Body-Vel/Fz drag1 ==
  data: vy input; Fy_d output
function Fy_d  = fcn(vy)
%#codegen
% v = max( 0.001,min(1,vy));
% i = round(v*1000);
% Fy_d = Fxy_drag(i);

% fitFxy = 
% 
%      General model:
%      fitFxy(x) = a*x^2 + b*x
%      Coefficients (with 95% confidence bounds):
%        a =   0.0002158  (0.0002153, 0.0002162)
%        b =   0.0005734  (0.0005717, 0.0005751)
       
if (vy >= 0)
%     Fy_d = 0.0002158.*vy.^2+0.0005734 .*vy;%+-7.949e-05;
     Fy_d = .5*(0.0002158.*vy.^2+0.0005734 .*vy);%+-7.949e-05;
else
    Fy_d = .5*(-(0.0002158.*vy.^2)+0.0005734 .*vy);%+-7.949e-05;
end

== matlab function iros2018_AoA/Plant/Dynamics/DRAG Body-Vel/Fxy drag2 ==
  data: vz input; Fz_d output
function Fz_d = fcn(vz)
%#codegen
% v = max( 0.001,min(1,vz));
% i = round(v*1000);
% Fz_d = Fz_drag(i);
% fitFz = 
% 
%      General model:
%      fitFz(x) = a*x^2 + b*x
%      Coefficients (with 95% confidence bounds):
%        a =   4.315e-07  (4.307e-07, 4.324e-07)
%        b =   1.147e-06  (1.143e-06, 1.15e-06)    

if (vz >=0)
    Fz_d = 4.315e-07.*vz.^2+1.147e-06.*vz;%+-1.59e-07;
else
    Fz_d = -(4.315e-07.*vz.^2)+1.147e-06.*vz;%+-1.59e-07;
end

== matlab function iros2018_AoA/Plant/Dynamics/DRAG Global Wind/Fxy drag1 ==
  data: vz input; Fz_d output
function Fz_d = fcn(vz)
%#codegen
% v = max( 0.001,min(1,vz));
% i = round(v*1000);
% Fz_d = Fz_drag(i);
% fitFz = 
% 
%      General model:
%      fitFz(x) = a*x^2 + b*x
%      Coefficients (with 95% confidence bounds):
%        a =   4.315e-07  (4.307e-07, 4.324e-07)
%        b =   1.147e-06  (1.143e-06, 1.15e-06)    

if (vz >=0)
    Fz_d = 4.315e-07.*vz.^2+1.147e-06.*vz;%+-1.59e-07;
else
    Fz_d = -(4.315e-07.*vz.^2)+1.147e-06.*vz;%+-1.59e-07;
end

== matlab function iros2018_AoA/Plant/Dynamics/DRAG Global Wind/Fxy drag2 ==
  data: vz input; Fz_d output
function Fz_d = fcn(vz)
%#codegen
% v = max( 0.001,min(1,vz));
% i = round(v*1000);
% Fz_d = Fz_drag(i);
% fitFz = 
% 
%      General model:
%      fitFz(x) = a*x^2 + b*x
%      Coefficients (with 95% confidence bounds):
%        a =   4.315e-07  (4.307e-07, 4.324e-07)
%        b =   1.147e-06  (1.143e-06, 1.15e-06)    

if (vz >=0)
    Fz_d = 4.315e-07.*vz.^2+1.147e-06.*vz;%+-1.59e-07;
else
    Fz_d = -(4.315e-07.*vz.^2)+1.147e-06.*vz;%+-1.59e-07;
end

== matlab function iros2018_AoA/Plant/Dynamics/DRAG Body-Vel/Projection Lift ==
  data: Vx input; F_lift_body output; Vy input; Vz input; y input; p input; r input; time input
function F_lift_body = fcn(Vx, Vy, Vz, y, p, r, time)
%#codegen
% Takes in body velocity vectors and returns global drag force vector
%       V_body = [vx, vy, vz]
%       Drag_body = f([vx, vy, vz]) 
%       [Fx, Fy, Fz] = f(drag_body, [yaw, pitch, roll])

% Drag is fit to:
%   f(theta,v) = (w1*theta+w2)*v^2+(w3*theta+w4)*v
%   w= [-0.07370093  0.09642926 -0.06727348  0.11939324]

% This approximation is only valid for small angles of attack, so theta is
% in the bounded region of [0,30] ish

% If needed: Fitting body drag vector to global is just the transformation of body to
% global with yaw pitch and roll

%% Grabs values for projections
if time == 0
    F_lift_body = [0,0,0];
else  
    
% Vb
% Vx = Vb(1);
% Vy = Vb(2);
% Vz = Vb(3);

w= [-0.0420483   0.03801497  0.59340685  0.00751537];

% yaw = attitude(1);
% pitch = attitude(2);
% roll = attitude(3);

% Extracts Angles
theta_yz = atan(Vz/Vy);
theta_xz = atan(Vz/Vx);

% Gets velocity number
v_yz = norm([Vy, Vz]);
v_xz = norm([Vx, Vz]);

% Computes Drag
F_d_yz = (w(1)*(theta_yz)+w(2))*v_yz^2 + (w(3)*(theta_yz)+w(4))*v_yz^2;
F_d_xz = (w(1)*(theta_xz)+w(2))*v_xz^2 + (w(3)*(theta_xz)+w(4))*v_xz^2;

% Vectorized drag output

F_d_yz_v = 1e-3.*[0, Vy/(Vy + Vz), .5*Vz/(Vy + Vz)] .* F_d_yz;
F_d_xz_v = 1e-3.*[Vx/(Vx + Vz), 0, .5*Vz/(Vx + Vz)] .* F_d_xz;

if theta_yz < 0
    F_d_yz_v = -1*F_d_yz_v;
end
if theta_xz < 0
    F_d_xz_v = -1*F_d_xz_v;
end
%{
%% Defines matrices for getting global forces
Ryaw = [
	[ cos(yaw), -sin(yaw), 0],
	[ sin(yaw),  cos(yaw), 0],
	[        0,         0, 1]
];

Rpitch = [
	[  cos(pitch), 0, sin(pitch)],
	[           0, 1,          0],
	[ -sin(pitch), 0, cos(pitch)]
];

Rroll = [
	[ 1,         0,          0],
	[ 0, cos(roll), -sin(roll)],
	[ 0, sin(roll),  cos(roll)]
];

Body2Global = Ryaw*Rpitch*Rroll;
%}
% F_drag_body = [0, 0, 0];
R_veltolift = [
        [0, 1, 0],
        [-1, 0, 0],
        [0, 0, 1]
];

F_lift_body = [F_d_xz_v(1), F_d_yz_v(2), F_d_xz_v(3)+F_d_yz_v(3)]*R_veltolift;

end 
% F_drag = Body2Global*F_drag_body;

== matlab function iros2018_AoA/Plant/Dynamics/DRAG Global Wind/Fz drag1 ==
  data: vy input; Fy_d output
function Fy_d  = fcn(vy)
%#codegen
% v = max( 0.001,min(1,vy));
% i = round(v*1000);
% Fy_d = Fxy_drag(i);

% fitFxy = 
% 
%      General model:
%      fitFxy(x) = a*x^2 + b*x
%      Coefficients (with 95% confidence bounds):
%        a =   0.0002158  (0.0002153, 0.0002162)
%        b =   0.0005734  (0.0005717, 0.0005751)
       
if (vy >= 0)
%     Fy_d = 0.0002158.*vy.^2+0.0005734 .*vy;%+-7.949e-05;
     Fy_d = .5*(0.0002158.*vy.^2+0.0005734 .*vy);%+-7.949e-05;
else
    Fy_d = .5*(-(0.0002158.*vy.^2)+0.0005734 .*vy);%+-7.949e-05;
end

== matlab function iros2018_AoA/Controller/Force Regulator/Force Correction/MATLAB Function ==
  data: u input; y output; maxF input; t input
function y = fcn(u, maxF,t) 
% u = [f4 f3 f2 f1]
 % Y = [f4 f3 f2 f1]
y = [0; 0; 0; 0;];          
for i = 1:4
   utemp = u(i);
   utemp = max(utemp,-0.0);        % eliminates negative forces
   utemp = min(maxF, utemp);     % reduces forces above the max
   y(i) = utemp;
end
if (t < .1)
    y(1:4) = maxF;
end

== matlab function iros2018_AoA/Plant/Dynamics/DRAG Body-Vel/Taux drag ==
  data: wx input; Taux_d output
function Taux_d = fcn(wx)
%#codegen
% v = max( 0.001,min(1,wx));
% i = round(v*1000);
% Taux_d = Taux_drag(i);

% fitTx = 
% 
%      General model:
%      fitTx(x) = a*x^2 + b*x
%      Coefficients (with 95% confidence bounds):
%        a =    7.49e-10  (7.41e-10, 7.569e-10)
%        b =   2.138e-09  (2.076e-09, 2.199e-09)

if (wx >=0)
    Taux_d = .5*(7.49e-10.*wx.^2+ 2.138e-09.*wx);%+ 2.759e-08;
else
    Taux_d = .5*(-(7.49e-10.*wx.^2)+ 2.138e-09.*wx);%+ 2.759e-08;
end

== matlab function iros2018_AoA/Plant/Dynamics/DRAG Body-Vel/Tauy drag ==
  data: wy input; Tauy_d output
function Tauy_d = fcn(wy)
%#codegen
% v = max(0.001,min(1,wy));
% i = round(v*1000);
% Tauy_d = Tauy_drag(i);
% 

% fitTy = 
% 
%      General model:
%      fitTy(x) = a*x^2 + b*x
%      Coefficients (with 95% confidence bounds):
%        a =    7.49e-10  (7.41e-10, 7.569e-10)
%        b =   2.138e-09  (2.076e-09, 2.199e-09)
        
if (wy >=0)
    Tauy_d =  .5*(7.49e-10.*wy.^2 + 2.138e-09.*wy);%+2.759e-08;
else
    Tauy_d =  .5*(-(7.49e-10.*wy.^2) + 2.138e-09.*wy);%+2.759e-08;
end

== matlab function iros2018_AoA/Plant/Dynamics/DRAG Body-Vel/Tauz drag ==
  data: wz input; Tauz_d output
function Tauz_d = fcn(wz)
%#codegen
% v = max( 0.001,min(1,wz));
% i = round(v*1000);
% Tauz_d = Tauz_drag(i);
% % 
% fitTz = 
% 
%      General model:
%      fitTz(x) = a*x^2 + b*x
%      Coefficients (with 95% confidence bounds):
%        a =   1.498e-12  (1.482e-12, 1.514e-12)
%        b =   4.275e-12  (4.152e-12, 4.398e-12)


if (wz >=0)
    Tauz_d = 1.498e-12.*wz.^2+ 4.275e-12.*wz;%+ 5.517e-11;
else
    Tauz_d = -(1.498e-12.*wz.^2)+ 4.275e-12.*wz;%+ 5.517e-11;
end
